simulink subsystem "SCIOutAbFOCSL"  (R2024b)
settings: Solver=VariableStepAuto  StartTime=0.0  StopTime=10.0  RelTol=1e-3
values from neighbouring files (symbols this model uses):
  dataType = 'single'    [s32k344Data.m]
undefined symbols (not defined in the file or in its folder): inverter
libraries: svdutilitieslib x1
settings Model: Creator=The MathWorks, Inc.  LastModifiedBy=snarayan
settings RTWCC: GPUComputeCapability=3.5

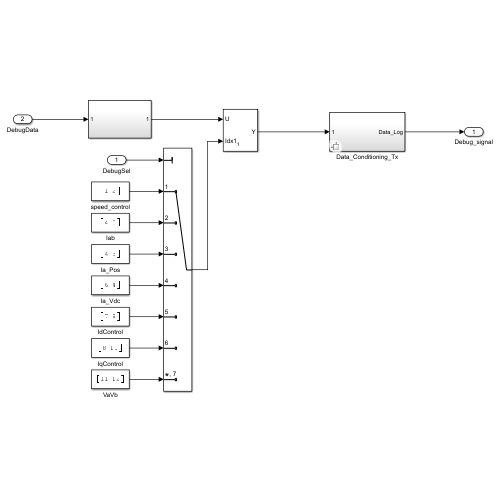
[thumbnail: Simulink's stored preview of the top-level diagram]
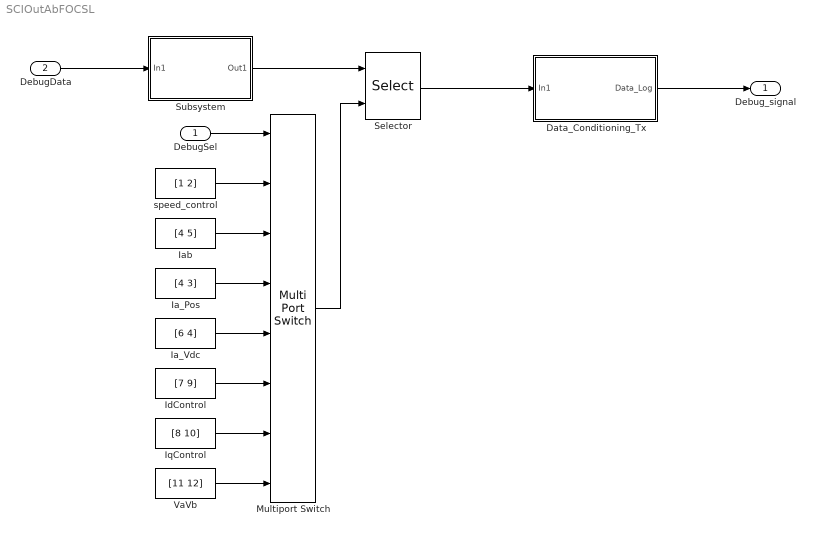
== system SCIOutAbFOCSL ==
  DebugSel : Inport
  DebugData : Inport  Port=2
  Data_Conditioning_Tx : Subsystem  Variant=on
  Ia_Pos : Constant  Value=[4 3]  OutDataTypeStr=uint16  SampleTime=-1
  Ia_Vdc : Constant  Value=[6 4]  OutDataTypeStr=uint16  SampleTime=-1
  Iab : Constant  Value=[4 5]  OutDataTypeStr=uint16  SampleTime=-1
  IdControl : Constant  Value=[7 9]  OutDataTypeStr=uint16  SampleTime=-1
  IqControl : Constant  Value=[8 10]  OutDataTypeStr=uint16  SampleTime=-1
  Multiport Switch : MultiPortSwitch  Inputs=7  DiagnosticForDefault=None  OutDataTypeStr=uint16  RndMeth=Simplest  SaturateOnIntegerOverflow=off  InputSameDT=off
  Selector : Selector  InputPortWidth=13  IndexOptions=Index vector (port)  Indices=[1 3]  OutputSizes=1
  Subsystem : Subsystem
  VaVb : Constant  Value=[11 12]  OutDataTypeStr=uint16  SampleTime=-1
  speed_control : Constant  Value=[1 2]  OutDataTypeStr=uint16  SampleTime=-1
  Debug_signal : Outport
  wires:
  speed_control/1 -> Multiport Switch/2
  Multiport Switch/1 -> Selector/2
  DebugSel/1 -> Multiport Switch/1
  Selector/1 -> Data_Conditioning_Tx/1(In1)
  Data_Conditioning_Tx/1(Data_Log) -> Debug_signal/1
  Iab/1 -> Multiport Switch/3
  Ia_Pos/1 -> Multiport Switch/4
  DebugData/1 -> Subsystem/1(In1)
  Subsystem/1(Out1) -> Selector/1
  Ia_Vdc/1 -> Multiport Switch/5
  IdControl/1 -> Multiport Switch/6
  IqControl/1 -> Multiport Switch/7
  VaVb/1 -> Multiport Switch/8

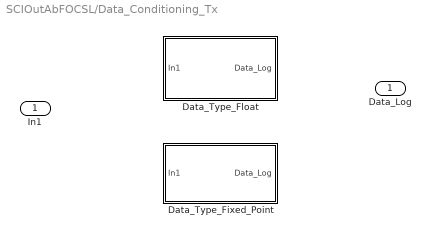
== system SCIOutAbFOCSL/Data_Conditioning_Tx ==
  In1 : Inport
  Data_Type_Fixed_Point : Subsystem  VariantControl=~isequal(dataType,'single')
  Data_Type_Float : Subsystem  VariantControl=isequal(dataType, 'single')
  Data_Log : Outport

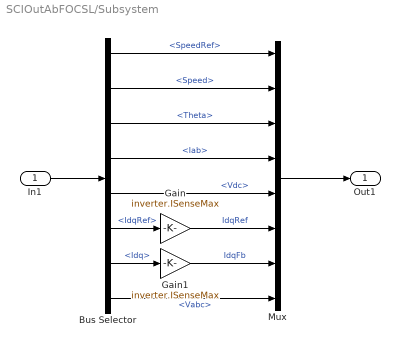
== system SCIOutAbFOCSL/Subsystem ==
  In1 : Inport
  Bus Selector : BusSelector  OutputSignals=SpeedRef,Speed,Theta,Iab,Vdc,IdqRef,Idq,Vabc
  Gain : Gain  Gain=inverter.ISenseMax  RndMeth=Simplest  OutDataTypeStr=Inherit: Same as input
  Gain1 : Gain  Gain=inverter.ISenseMax  RndMeth=Simplest  OutDataTypeStr=Inherit: Same as input
  Mux : Mux  Inputs=8
  Out1 : Outport
  wires:
  Gain1/1 -> Mux/7  "IdqFb"
  Gain/1 -> Mux/6  "IdqRef"
  Bus Selector/8 -> Mux/8  "<Vabc>"
  Bus Selector/7 -> Gain1/1  "<Idq>"
  Bus Selector/6 -> Gain/1  "<IdqRef>"
  Bus Selector/5 -> Mux/5  "<Vdc>"
  Mux/1 -> Out1/1
  In1/1 -> Bus Selector/1
  Bus Selector/3 -> Mux/3  "<Theta>"
  Bus Selector/1 -> Mux/1  "<SpeedRef>"
  Bus Selector/4 -> Mux/4  "<Iab>"
  Bus Selector/2 -> Mux/2  "<Speed>"

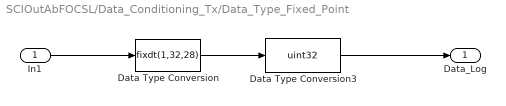
== system SCIOutAbFOCSL/Data_Conditioning_Tx/Data_Type_Fixed_Point ==
  In1 : Inport
  Data Type Conversion : DataTypeConversion  OutDataTypeStr=fixdt(1,32,28)  RndMeth=Simplest  SaturateOnIntegerOverflow=off
  Data Type Conversion3 : DataTypeConversion  OutDataTypeStr=uint32  ConvertRealWorld=Stored Integer (SI)  RndMeth=Simplest  SaturateOnIntegerOverflow=off
  Data_Log : Outport
  wires:
  Data Type Conversion/1 -> Data Type Conversion3/1
  Data Type Conversion3/1 -> Data_Log/1
  In1/1 -> Data Type Conversion/1

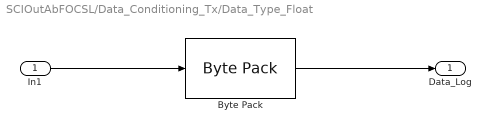
== system SCIOutAbFOCSL/Data_Conditioning_Tx/Data_Type_Float ==
  In1 : Inport
  Byte Pack : svdutilitieslib/Byte Pack  maskPackedDataType=uint8  datatypes={'single'}  byteAlign=4  blockPlatform=tic2000
  Data_Log : Outport
  wires:
  In1/1 -> Byte Pack/1
  Byte Pack/1 -> Data_Log/1
